simulink model "PE_V2_0"  (R2020b)
settings: Solver=VariableStepAuto  StartTime=0.0  StopTime=10.0  RelTol=1e-3
undefined symbols (not defined in the file): ZERO
libraries: hdlsllib x35, simulink x28, visionhdlutilities x12
(part 3 of 3)

== system PE_V2_0/2DCov PEV1.1/MaxPooling/OutValidGen ==
  ctrl : Inport
  Window_Width : Inport  Port=2
  Feature_Height : Inport  Port=3
  Compare To Constant : simulink/Logic and Bit Operations/Compare To Constant  Commented=on  relop=>  const=0  OutDataTypeStr=boolean
  Constant : Constant  OutDataTypeStr=uint32  SampleTime=-1
  Delay36 : Delay  DelayLength=1
  Logical Operator1 : Logic  Operator=NOT  AllPortsSameDT=off  OutDataTypeStr=boolean
  Logical Operator3 : Logic  Inputs=3  AllPortsSameDT=off  OutDataTypeStr=boolean
  Logical Operator4 : Logic  Operator=NOT  AllPortsSameDT=off  OutDataTypeStr=boolean
  Logical Operator5 : Logic  Operator=OR  AllPortsSameDT=off  OutDataTypeStr=boolean
  Logical Operator6 : Logic  Operator=NOT  Inputs=3  AllPortsSameDT=off  OutDataTypeStr=boolean
  Minus1 : Sum  Inputs=+-
  Minus2 : Sum  Inputs=+-
  NumRow_Counter : hdlsllib/Sources/HDL Counter  CountType=Free running  CountInit=0  CountStep=1  CountMax=2^15  CountFromType=Initial value  CountFrom=0  CountResetPort=on  CountLoadPort=off  CountEnbPort=on  CountDirPort=off  CountDataType=Unsigned  CountWordLen=32  CountFracLen=0  CountSampTime=1
  Pixel Control Bus Selector : BusSelector  OutputSignals=hStart,hEnd,vStart,vEnd,valid
  Relational Operator1 : RelationalOperator  Operator=<  OutDataTypeStr=boolean  RndMeth=Nearest
  Relational Operator2 : RelationalOperator  Operator=<=  OutDataTypeStr=boolean  RndMeth=Nearest
  Row_Counter : hdlsllib/Sources/HDL Counter  CountType=Free running  CountInit=0  CountStep=1  CountMax=2^15  CountFromType=Initial value  CountFrom=0  CountResetPort=on  CountLoadPort=off  CountEnbPort=on  CountDirPort=off  CountDataType=Unsigned  CountWordLen=32  CountFracLen=0  CountSampTime=1
  Terminator1 : Terminator
  Out1 : Outport
  wires:
  NumRow_Counter/1 -> Relational Operator2/2, Compare To Constant/1
  Pixel Control Bus Selector/1 -> NumRow_Counter/2  "<hStart>"
  Minus2/1 -> Relational Operator2/1
  Relational Operator1/1 -> Logical Operator4/1
  Pixel Control Bus Selector/3 -> Logical Operator5/1  "<vStart>"
  Feature_Height/1 -> Minus2/1
  Minus1/1 -> Relational Operator1/2
  Row_Counter/1 -> Relational Operator1/1
  Pixel Control Bus Selector/5 -> Row_Counter/2, Logical Operator1/1, Logical Operator3/2  "<valid>"
  Window_Width/1 -> Minus1/1
  Pixel Control Bus Selector/2 -> Terminator1/1  "<hEnd>"
  Delay36/1 -> Pixel Control Bus Selector/1
  Constant/1 -> Minus1/2, Minus2/2
  Logical Operator6/1 -> Logical Operator3/1
  Logical Operator5/1 -> NumRow_Counter/1
  Pixel Control Bus Selector/4 -> Logical Operator5/2  "<vEnd>"
  Relational Operator2/1 -> Logical Operator6/1
  Logical Operator1/1 -> Row_Counter/1
  Logical Operator4/1 -> Logical Operator3/3
  Logical Operator3/1 -> Out1/1
  ctrl/1 -> Delay36/1

== system PE_V2_0/2DCov PEV1.1/MaxPooling/window Selector ==
  pixel : Inport
  valid : Inport  Port=2
  step : Inport  Port=3
  Add : Sum  Inputs=+-
  Compare To Zero : simulink/Logic and Bit Operations/Compare To Zero  relop===  OutDataTypeStr=boolean
  Constant : Constant  OutDataTypeStr=uint32
  Delay : Delay
  Delay1 : Delay  DelayLength=1
  Delay36 : Delay  DelayLength=1
  Logical Operator : Logic  Operator=NOT  AllPortsSameDT=off  OutDataTypeStr=boolean
  Logical Operator1 : Logic  Operator=OR  AllPortsSameDT=off  OutDataTypeStr=boolean
  Logical Operator2 : Logic  AllPortsSameDT=off  OutDataTypeStr=boolean
  Relational Operator : RelationalOperator  OutDataTypeStr=boolean  RndMeth=Nearest
  Selector1 : Selector  InputPortWidth=2  IndexOptions=Index vector (dialog)  Indices=[1]  OutputSizes=1
  Selector2 : Selector  InputPortWidth=2  IndexOptions=Index vector (dialog)  Indices=[2]  OutputSizes=1
  Selector3 : Selector  InputPortWidth=2  IndexOptions=Index vector (dialog)  Indices=[1]  OutputSizes=1
  Selector4 : Selector  InputPortWidth=2  IndexOptions=Index vector (dialog)  Indices=[2]  OutputSizes=1
  Step Counter : hdlsllib/Sources/HDL Counter  CountType=Free running  CountInit=0  CountStep=1  CountMax=2^15  CountFromType=Initial value  CountFrom=0  CountResetPort=on  CountLoadPort=off  CountEnbPort=on  CountDirPort=off  CountDataType=Unsigned  CountWordLen=32  CountFracLen=0  CountSampTime=1
  Out1 : Outport
  Out2 : Outport  Port=2
  Out3 : Outport  Port=3
  Out4 : Outport  Port=4
  Valid : Outport  Port=5
  wires:
  Selector2/1 -> Out2/1
  Delay/1 -> Selector4/1, Selector3/1
  Selector3/1 -> Out3/1
  Selector1/1 -> Out1/1
  Selector4/1 -> Out4/1
  pixel/1 -> Delay36/1, Delay/1
  Step Counter/1 -> Compare To Zero/1, Relational Operator/1
  Delay1/1 -> Logical Operator2/2, Step Counter/2, Logical Operator/1
  Logical Operator/1 -> Logical Operator1/2
  step/1 -> Add/1
  Constant/1 -> Add/2
  Add/1 -> Relational Operator/2
  Relational Operator/1 -> Logical Operator1/1
  Logical Operator1/1 -> Step Counter/1
  Compare To Zero/1 -> Logical Operator2/1
  Logical Operator2/1 -> Valid/1
  Delay36/1 -> Selector2/1, Selector1/1
  valid/1 -> Delay1/1

== system PE_V2_0/2DConvPE1 V1.5/FUNCTION/Subsystem1/LIne Buffer ==
  Stream_In : Inport
  Stream_Valid : Inport  Port=2
  Weight_Width : Inport  Port=3
  Feature_Area : Inport  Port=4
  Feature_Width : Inport  Port=5
  Feature_Height : Inport  Port=6
  Delay2 : Delay  DelayLength=1
  Line Buffer : Subsystem
  OutValidGen : Subsystem
  Terminator : Terminator
  pixel : Outport
  valid : Outport  Port=2
  wires:
  Feature_Area/1 -> Line Buffer/3(Feature_Area)
  Feature_Height/1 -> OutValidGen/3(Feature_Height)
  Line Buffer/3(shftEnable) -> Terminator/1
  Stream_In/1 -> Line Buffer/1(Stream_In)
  Line Buffer/1(pixel) -> Delay2/1
  Line Buffer/2(ctrl) -> OutValidGen/1(In1)
  Feature_Width/1 -> Line Buffer/4(Feature_Width)
  Stream_Valid/1 -> Line Buffer/2(Stream_Valid)
  Weight_Width/1 -> OutValidGen/2(Weight_Width)
  OutValidGen/1(valid) -> valid/1
  Delay2/1 -> pixel/1

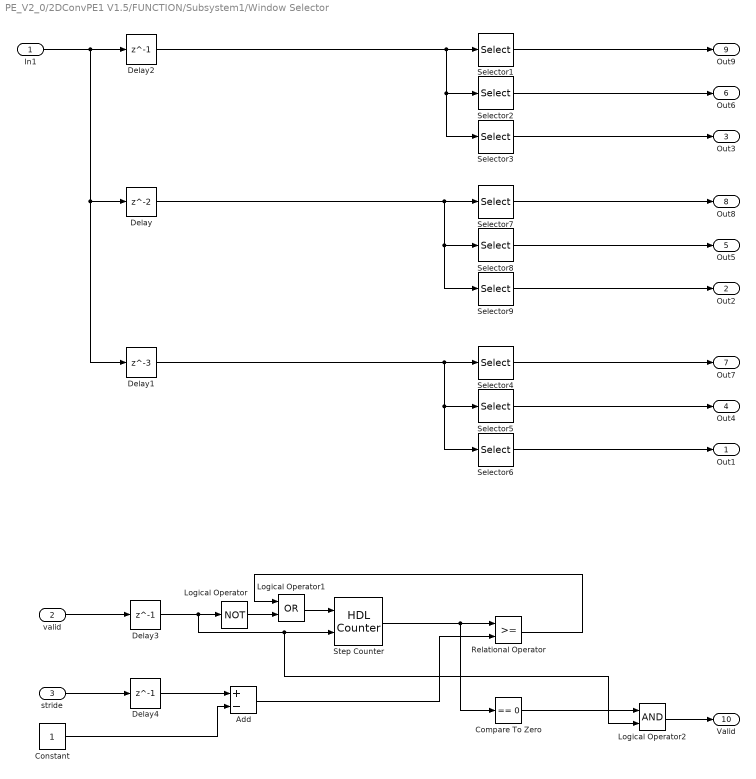
== system PE_V2_0/2DConvPE1 V1.5/FUNCTION/Subsystem1/Window Selector ==
  In1 : Inport
  valid : Inport  Port=2
  stride : Inport  Port=3
  Add : Sum  Inputs=+-
  Compare To Zero : simulink/Logic and Bit Operations/Compare To Zero  relop===  OutDataTypeStr=boolean
  Constant : Constant  OutDataTypeStr=uint32
  Delay : Delay
  Delay1 : Delay  DelayLength=3
  Delay2 : Delay  DelayLength=1
  Delay3 : Delay  DelayLength=1
  Delay4 : Delay  DelayLength=1
  Logical Operator : Logic  Operator=NOT  AllPortsSameDT=off  OutDataTypeStr=boolean
  Logical Operator1 : Logic  Operator=OR  AllPortsSameDT=off  OutDataTypeStr=boolean
  Logical Operator2 : Logic  AllPortsSameDT=off  OutDataTypeStr=boolean
  Relational Operator : RelationalOperator  OutDataTypeStr=boolean  RndMeth=Nearest
  Selector1 : Selector  InputPortWidth=3  IndexOptions=Index vector (dialog)  Indices=[1]  OutputSizes=1
  Selector2 : Selector  InputPortWidth=3  IndexOptions=Index vector (dialog)  Indices=[2]  OutputSizes=1
  Selector3 : Selector  InputPortWidth=3  IndexOptions=Index vector (dialog)  Indices=[3]  OutputSizes=1
  Selector4 : Selector  InputPortWidth=3  IndexOptions=Index vector (dialog)  Indices=[1]  OutputSizes=1
  Selector5 : Selector  InputPortWidth=3  IndexOptions=Index vector (dialog)  Indices=[2]  OutputSizes=1
  Selector6 : Selector  InputPortWidth=3  IndexOptions=Index vector (dialog)  Indices=[3]  OutputSizes=1
  Selector7 : Selector  InputPortWidth=3  IndexOptions=Index vector (dialog)  Indices=[1]  OutputSizes=1
  Selector8 : Selector  InputPortWidth=3  IndexOptions=Index vector (dialog)  Indices=[2]  OutputSizes=1
  Selector9 : Selector  InputPortWidth=3  IndexOptions=Index vector (dialog)  Indices=[3]  OutputSizes=1
  Step Counter : hdlsllib/Sources/HDL Counter  CountType=Free running  CountInit=0  CountStep=1  CountMax=2^15  CountFromType=Initial value  CountFrom=0  CountResetPort=on  CountLoadPort=off  CountEnbPort=on  CountDirPort=off  CountDataType=Unsigned  CountWordLen=32  CountFracLen=0  CountSampTime=1
  Out1 : Outport
  Out2 : Outport  Port=2
  Out3 : Outport  Port=3
  Out4 : Outport  Port=4
  Out5 : Outport  Port=5
  Out6 : Outport  Port=6
  Out7 : Outport  Port=7
  Out8 : Outport  Port=8
  Out9 : Outport  Port=9
  Valid : Outport  Port=10
  wires:
  In1/1 -> Delay2/1, Delay1/1, Delay/1
  Selector9/1 -> Out2/1
  Delay/1 -> Selector9/1, Selector8/1, Selector7/1
  Selector5/1 -> Out4/1
  Selector6/1 -> Out1/1
  Selector4/1 -> Out7/1
  Delay1/1 -> Selector6/1, Selector5/1, Selector4/1
  Relational Operator/1 -> Logical Operator1/1
  Constant/1 -> Add/2
  Logical Operator2/1 -> Valid/1
  Compare To Zero/1 -> Logical Operator2/1
  Logical Operator1/1 -> Step Counter/1
  Logical Operator/1 -> Logical Operator1/2
  Delay4/1 -> Add/1
  Step Counter/1 -> Compare To Zero/1, Relational Operator/1
  Delay3/1 -> Logical Operator2/2, Step Counter/2, Logical Operator/1
  Add/1 -> Relational Operator/2
  Delay2/1 -> Selector3/1, Selector2/1, Selector1/1
  valid/1 -> Delay3/1
  stride/1 -> Delay4/1
  Selector8/1 -> Out5/1
  Selector7/1 -> Out8/1
  Selector3/1 -> Out3/1
  Selector2/1 -> Out6/1
  Selector1/1 -> Out9/1

== system PE_V2_0/2DConvPE1 V1.5/FUNCTION/Subsystem1/weight_register ==
  In1 : Inport
  Enable : EnablePort
  Delay{1,3..8,40} (8 alike) : Delay  DelayLength=1
  Out2 : Outport
  Out3 : Outport  Port=2
  Out4 : Outport  Port=3
  Out5 : Outport  Port=4
  Out6 : Outport  Port=5
  Out7 : Outport  Port=6
  Out8 : Outport  Port=7
  Out9 : Outport  Port=8
  Out1 : Outport  Port=9
  wires:
  Delay40/1 -> Delay7/1, Out9/1
  In1/1 -> Out1/1, Delay40/1
  Delay7/1 -> Out8/1, Delay1/1
  Delay1/1 -> Out7/1, Delay5/1
  Delay5/1 -> Out6/1, Delay8/1
  Delay8/1 -> Out5/1, Delay6/1
  Delay6/1 -> Out4/1, Delay4/1
  Delay4/1 -> Out3/1, Delay3/1
  Delay3/1 -> Out2/1

== system PE_V2_0/2DConvPE1 V1.5/MaxPooling/Line Buffer1/CtrlGen ==
  note: valid
  note: vEnd
  note: vStart
  note: hEnd
  note: hstart
  Stream_In : Inport
  Stream_Valid : Inport  Port=2
  Feature_Area : Inport  Port=3
  Feature_Width : Inport  Port=4
  Compare To Zero : simulink/Logic and Bit Operations/Compare To Zero  relop===  OutDataTypeStr=boolean
  Compare To Zero1 : simulink/Logic and Bit Operations/Compare To Zero  relop===  OutDataTypeStr=boolean
  Constant : Constant  OutDataTypeStr=uint32  SampleTime=-1
  Constant1 : Constant  OutDataTypeStr=uint32  SampleTime=-1
  Delay1 : Delay  DelayLength=1
  Delay36 : Delay  DelayLength=1
  Feature Area Counter : hdlsllib/Sources/HDL Counter  CountType=Free running  CountInit=0  CountStep=1  CountMax=2^15  CountFromType=Initial value  CountFrom=0  CountResetPort=on  CountLoadPort=off  CountEnbPort=on  CountDirPort=off  CountDataType=Unsigned  CountWordLen=32  CountFracLen=0  CountSampTime=1
  Feature Row Counter : hdlsllib/Sources/HDL Counter  CountType=Free running  CountInit=0  CountStep=1  CountMax=2^15  CountFromType=Initial value  CountFrom=0  CountResetPort=on  CountLoadPort=off  CountEnbPort=on  CountDirPort=off  CountDataType=Unsigned  CountWordLen=32  CountFracLen=0  CountSampTime=1
  Logical Operator : Logic  Operator=OR  AllPortsSameDT=off  OutDataTypeStr=boolean
  Logical Operator{1..3,5} (4 alike) : Logic  AllPortsSameDT=off  OutDataTypeStr=boolean
  Minus1 : Sum  Inputs=+-
  Minus2 : Sum  Inputs=+-
  Pixel Control Bus Creator : visionhdlutilities/Pixel Control Bus Creator
      settings: SourceProductBaseCode=VT
  Relational Operator1 : RelationalOperator  Operator===  OutDataTypeStr=boolean  RndMeth=Nearest
  Relational Operator2 : RelationalOperator  Operator===  OutDataTypeStr=boolean  RndMeth=Nearest
  Relational Operator3 : RelationalOperator  Operator===  OutDataTypeStr=boolean  RndMeth=Nearest
  StreamOut : Outport
  Ctrl : Outport  Port=2
  wires:
  Minus2/1 -> Relational Operator3/2, Relational Operator2/2
  Feature Row Counter/1 -> Relational Operator2/1, Relational Operator3/1, Compare To Zero/1
  Relational Operator2/1 -> Feature Row Counter/1
  Compare To Zero/1 -> Logical Operator/2
  Relational Operator3/1 -> Logical Operator2/1
  Feature_Area/1 -> Minus1/1
  Constant/1 -> Minus1/2
  Logical Operator/1 -> Logical Operator1/1
  Constant1/1 -> Minus2/2
  Feature_Width/1 -> Minus2/1
  Pixel Control Bus Creator/1 -> Ctrl/1
  Delay1/1 -> Feature Area Counter/2, Feature Row Counter/2, Logical Operator5/2, Logical Operator2/2, Logical Operator1/2, Logical Operator3/2, Pixel Control Bus Creator/5
  Delay36/1 -> StreamOut/1
  Logical Operator1/1 -> Pixel Control Bus Creator/1
  Logical Operator2/1 -> Pixel Control Bus Creator/2
  Logical Operator3/1 -> Pixel Control Bus Creator/4
  Logical Operator5/1 -> Pixel Control Bus Creator/3
  Feature Area Counter/1 -> Compare To Zero1/1, Relational Operator1/1
  Minus1/1 -> Relational Operator1/2
  Relational Operator1/1 -> Feature Area Counter/1, Logical Operator3/1
  Compare To Zero1/1 -> Logical Operator/1, Logical Operator5/1
  Stream_In/1 -> Delay36/1
  Stream_Valid/1 -> Delay1/1

== system PE_V2_0/2DConvPE1 V2.0/Line Buffer/LIne Buffer/Line Buffer ==
  Stream_In : Inport
  Stream_Valid : Inport  Port=2
  Feature_Area : Inport  Port=3
  Feature_Width : Inport  Port=4
  CtrlGen : Subsystem
  Line Buffer : visionhdlutilities/Line Buffer  NeighborhoodSize=[3 1]  PaddingMethod=Constant  PaddingValue=0  LineBufferSize=128  SimulateUsing=Code generation
      settings: SourceProductBaseCode=VT
  pixel : Outport
  ctrl : Outport  Port=2
  shftEnable : Outport  Port=3
  wires:
  Feature_Area/1 -> CtrlGen/3(Feature_Area)
  Line Buffer/2 -> ctrl/1
  CtrlGen/1(StreamOut) -> Line Buffer/1
  Feature_Width/1 -> CtrlGen/4(Feature_Width)
  Stream_In/1 -> CtrlGen/1(Stream_In)
  CtrlGen/2(Ctrl) -> Line Buffer/2
  Stream_Valid/1 -> CtrlGen/2(Stream_Valid)
  Line Buffer/3 -> shftEnable/1
  Line Buffer/1 -> pixel/1

== system PE_V2_0/2DConvPE1 V2.0/Line Buffer/LIne Buffer/OutValidGen ==
  In1 : Inport
  Weight_Width : Inport  Port=2
  Feature_Height : Inport  Port=3
  Compare To Constant : simulink/Logic and Bit Operations/Compare To Constant  relop=>  const=0  OutDataTypeStr=boolean
  Constant : Constant  OutDataTypeStr=uint32  SampleTime=-1
  Delay2 : Delay  DelayLength=1
  Logical Operator1 : Logic  Operator=NOT  AllPortsSameDT=off  OutDataTypeStr=boolean
  Logical Operator2 : Logic  Operator=OR  AllPortsSameDT=off  OutDataTypeStr=boolean
  Logical Operator3 : Logic  Inputs=4  AllPortsSameDT=off  OutDataTypeStr=boolean
  Logical Operator4 : Logic  Operator=NOT  AllPortsSameDT=off  OutDataTypeStr=boolean
  Logical Operator5 : Logic  Operator=OR  AllPortsSameDT=off  OutDataTypeStr=boolean
  Logical Operator6 : Logic  Operator=NOT  Inputs=3  AllPortsSameDT=off  OutDataTypeStr=boolean
  Minus1 : Sum  Inputs=+--
  Minus2 : Sum  Inputs=+-
  NumRow_Counter : hdlsllib/Sources/HDL Counter  CountType=Free running  CountInit=0  CountStep=1  CountMax=2^15  CountFromType=Initial value  CountFrom=0  CountResetPort=on  CountLoadPort=off  CountEnbPort=on  CountDirPort=off  CountDataType=Unsigned  CountWordLen=32  CountFracLen=0  CountSampTime=1
  Pixel Control Bus Selector : BusSelector  OutputSignals=hStart,hEnd,vStart,vEnd,valid
  Relational Operator1 : RelationalOperator  Operator=<  OutDataTypeStr=boolean  RndMeth=Nearest
  Relational Operator2 : RelationalOperator  Operator=<=  OutDataTypeStr=boolean  RndMeth=Nearest
  Row_Counter : hdlsllib/Sources/HDL Counter  CountType=Free running  CountInit=0  CountStep=1  CountMax=2^15  CountFromType=Initial value  CountFrom=0  CountResetPort=on  CountLoadPort=off  CountEnbPort=on  CountDirPort=off  CountDataType=Unsigned  CountWordLen=32  CountFracLen=0  CountSampTime=1
  Terminator1 : Terminator
  valid : Outport
  wires:
  Compare To Constant/1 -> Logical Operator3/2
  NumRow_Counter/1 -> Relational Operator2/2, Compare To Constant/1
  Pixel Control Bus Selector/1 -> NumRow_Counter/2, Logical Operator2/1  "<hStart>"
  Minus2/1 -> Relational Operator2/1
  Relational Operator1/1 -> Logical Operator4/1
  Logical Operator1/1 -> Logical Operator2/2
  Pixel Control Bus Selector/3 -> Logical Operator5/1  "<vStart>"
  Feature_Height/1 -> Minus2/1
  Minus1/1 -> Relational Operator1/2
  Row_Counter/1 -> Relational Operator1/1
  Pixel Control Bus Selector/5 -> Logical Operator1/1, Row_Counter/2, Logical Operator3/3  "<valid>"
  Weight_Width/1 -> Minus1/1
  Pixel Control Bus Selector/2 -> Terminator1/1  "<hEnd>"
  Delay2/1 -> Pixel Control Bus Selector/1
  Constant/1 -> Minus1/3, Minus1/2, Minus2/2
  Logical Operator6/1 -> Logical Operator3/1
  Logical Operator5/1 -> NumRow_Counter/1
  Pixel Control Bus Selector/4 -> Logical Operator5/2  "<vEnd>"
  Relational Operator2/1 -> Logical Operator6/1
  Logical Operator2/1 -> Row_Counter/1
  Logical Operator4/1 -> Logical Operator3/4
  Logical Operator3/1 -> valid/1
  In1/1 -> Delay2/1

== system PE_V2_0/2DConvPE1 V2.0/MaxPooling/Line Buffer1/CtrlGen ==
  note: valid
  note: vEnd
  note: vStart
  note: hEnd
  note: hstart
  Stream_In : Inport
  Stream_Valid : Inport  Port=2
  Feature_Area : Inport  Port=3
  Feature_Width : Inport  Port=4
  Compare To Zero : simulink/Logic and Bit Operations/Compare To Zero  relop===  OutDataTypeStr=boolean
  Compare To Zero1 : simulink/Logic and Bit Operations/Compare To Zero  relop===  OutDataTypeStr=boolean
  Constant : Constant  OutDataTypeStr=uint32  SampleTime=-1
  Constant1 : Constant  OutDataTypeStr=uint32  SampleTime=-1
  Delay1 : Delay  DelayLength=1
  Delay36 : Delay  DelayLength=1
  Feature Area Counter : hdlsllib/Sources/HDL Counter  CountType=Free running  CountInit=0  CountStep=1  CountMax=2^15  CountFromType=Initial value  CountFrom=0  CountResetPort=on  CountLoadPort=off  CountEnbPort=on  CountDirPort=off  CountDataType=Unsigned  CountWordLen=32  CountFracLen=0  CountSampTime=1
  Feature Row Counter : hdlsllib/Sources/HDL Counter  CountType=Free running  CountInit=0  CountStep=1  CountMax=2^15  CountFromType=Initial value  CountFrom=0  CountResetPort=on  CountLoadPort=off  CountEnbPort=on  CountDirPort=off  CountDataType=Unsigned  CountWordLen=32  CountFracLen=0  CountSampTime=1
  Logical Operator : Logic  Operator=OR  AllPortsSameDT=off  OutDataTypeStr=boolean
  Logical Operator{1..3,5} (4 alike) : Logic  AllPortsSameDT=off  OutDataTypeStr=boolean
  Minus1 : Sum  Inputs=+-
  Minus2 : Sum  Inputs=+-
  Pixel Control Bus Creator : visionhdlutilities/Pixel Control Bus Creator
      settings: SourceProductBaseCode=VT
  Relational Operator1 : RelationalOperator  Operator===  OutDataTypeStr=boolean  RndMeth=Nearest
  Relational Operator2 : RelationalOperator  Operator===  OutDataTypeStr=boolean  RndMeth=Nearest
  Relational Operator3 : RelationalOperator  Operator===  OutDataTypeStr=boolean  RndMeth=Nearest
  StreamOut : Outport
  Ctrl : Outport  Port=2
  wires:
  Minus2/1 -> Relational Operator3/2, Relational Operator2/2
  Feature Row Counter/1 -> Relational Operator2/1, Relational Operator3/1, Compare To Zero/1
  Relational Operator2/1 -> Feature Row Counter/1
  Compare To Zero/1 -> Logical Operator/2
  Relational Operator3/1 -> Logical Operator2/1
  Feature_Area/1 -> Minus1/1
  Constant/1 -> Minus1/2
  Logical Operator/1 -> Logical Operator1/1
  Constant1/1 -> Minus2/2
  Feature_Width/1 -> Minus2/1
  Pixel Control Bus Creator/1 -> Ctrl/1
  Delay1/1 -> Feature Area Counter/2, Feature Row Counter/2, Logical Operator5/2, Logical Operator2/2, Logical Operator1/2, Logical Operator3/2, Pixel Control Bus Creator/5
  Delay36/1 -> StreamOut/1
  Logical Operator1/1 -> Pixel Control Bus Creator/1
  Logical Operator2/1 -> Pixel Control Bus Creator/2
  Logical Operator3/1 -> Pixel Control Bus Creator/4
  Logical Operator5/1 -> Pixel Control Bus Creator/3
  Feature Area Counter/1 -> Compare To Zero1/1, Relational Operator1/1
  Minus1/1 -> Relational Operator1/2
  Relational Operator1/1 -> Feature Area Counter/1, Logical Operator3/1
  Compare To Zero1/1 -> Logical Operator/1, Logical Operator5/1
  Stream_In/1 -> Delay36/1
  Stream_Valid/1 -> Delay1/1

== system PE_V2_0/2DCov PEV1.1/LIne Buffer/Line Buffer/CtrlGen ==
  note: valid
  note: vEnd
  note: vStart
  note: hEnd
  note: hstart
  Stream_In : Inport
  Stream_Valid : Inport  Port=2
  Feature_Area : Inport  Port=3
  Feature_Width : Inport  Port=4
  Compare To Zero : simulink/Logic and Bit Operations/Compare To Zero  relop===  OutDataTypeStr=boolean
  Compare To Zero1 : simulink/Logic and Bit Operations/Compare To Zero  relop===  OutDataTypeStr=boolean
  Constant : Constant  OutDataTypeStr=uint32  SampleTime=-1
  Constant1 : Constant  OutDataTypeStr=uint32  SampleTime=-1
  Delay3 : Delay  DelayLength=1
  Delay35 : Delay  DelayLength=1
  Feature Area Counter : hdlsllib/Sources/HDL Counter  CountType=Free running  CountInit=0  CountStep=1  CountMax=2^15  CountFromType=Initial value  CountFrom=0  CountResetPort=on  CountLoadPort=off  CountEnbPort=on  CountDirPort=off  CountDataType=Unsigned  CountWordLen=32  CountFracLen=0  CountSampTime=1
  Feature Row Counter : hdlsllib/Sources/HDL Counter  CountType=Free running  CountInit=0  CountStep=1  CountMax=2^15  CountFromType=Initial value  CountFrom=0  CountResetPort=on  CountLoadPort=off  CountEnbPort=on  CountDirPort=off  CountDataType=Unsigned  CountWordLen=32  CountFracLen=0  CountSampTime=1
  Logical Operator : Logic  Operator=OR  AllPortsSameDT=off  OutDataTypeStr=boolean
  Logical Operator{1..3,5} (4 alike) : Logic  AllPortsSameDT=off  OutDataTypeStr=boolean
  Minus1 : Sum  Inputs=+-
  Minus2 : Sum  Inputs=+-
  Pixel Control Bus Creator : visionhdlutilities/Pixel Control Bus Creator
      settings: SourceProductBaseCode=VT
  Relational Operator1 : RelationalOperator  Operator===  OutDataTypeStr=boolean  RndMeth=Nearest
  Relational Operator2 : RelationalOperator  Operator===  OutDataTypeStr=boolean  RndMeth=Nearest
  Relational Operator3 : RelationalOperator  Operator===  OutDataTypeStr=boolean  RndMeth=Nearest
  StreamOut : Outport
  Ctrl : Outport  Port=2
  wires:
  Minus2/1 -> Relational Operator3/2, Relational Operator2/2
  Feature Row Counter/1 -> Relational Operator2/1, Relational Operator3/1, Compare To Zero/1
  Relational Operator2/1 -> Feature Row Counter/1
  Compare To Zero/1 -> Logical Operator/2
  Relational Operator3/1 -> Logical Operator2/1
  Feature_Area/1 -> Minus1/1
  Constant/1 -> Minus1/2
  Logical Operator/1 -> Logical Operator1/1
  Constant1/1 -> Minus2/2
  Feature_Width/1 -> Minus2/1
  Pixel Control Bus Creator/1 -> Ctrl/1
  Delay3/1 -> Feature Area Counter/2, Feature Row Counter/2, Logical Operator5/2, Logical Operator2/2, Logical Operator1/2, Logical Operator3/2, Pixel Control Bus Creator/5
  Stream_In/1 -> Delay35/1
  Logical Operator1/1 -> Pixel Control Bus Creator/1
  Logical Operator2/1 -> Pixel Control Bus Creator/2
  Logical Operator3/1 -> Pixel Control Bus Creator/4
  Logical Operator5/1 -> Pixel Control Bus Creator/3
  Feature Area Counter/1 -> Compare To Zero1/1, Relational Operator1/1
  Minus1/1 -> Relational Operator1/2
  Relational Operator1/1 -> Feature Area Counter/1, Logical Operator3/1
  Compare To Zero1/1 -> Logical Operator/1, Logical Operator5/1
  Delay35/1 -> StreamOut/1
  Stream_Valid/1 -> Delay3/1

== system PE_V2_0/2DCov PEV1.1/MaxPooling/Line Buffer1/CtrlGen ==
  note: valid
  note: vEnd
  note: vStart
  note: hEnd
  note: hstart
  Stream_In : Inport
  Stream_Valid : Inport  Port=2
  Feature_Area : Inport  Port=3
  Feature_Width : Inport  Port=4
  Compare To Zero : simulink/Logic and Bit Operations/Compare To Zero  relop===  OutDataTypeStr=boolean
  Compare To Zero1 : simulink/Logic and Bit Operations/Compare To Zero  relop===  OutDataTypeStr=boolean
  Constant : Constant  OutDataTypeStr=uint32  SampleTime=-1
  Constant1 : Constant  OutDataTypeStr=uint32  SampleTime=-1
  Delay1 : Delay  DelayLength=1
  Delay36 : Delay  DelayLength=1
  Feature Area Counter : hdlsllib/Sources/HDL Counter  CountType=Free running  CountInit=0  CountStep=1  CountMax=2^15  CountFromType=Initial value  CountFrom=0  CountResetPort=on  CountLoadPort=off  CountEnbPort=on  CountDirPort=off  CountDataType=Unsigned  CountWordLen=32  CountFracLen=0  CountSampTime=1
  Feature Row Counter : hdlsllib/Sources/HDL Counter  CountType=Free running  CountInit=0  CountStep=1  CountMax=2^15  CountFromType=Initial value  CountFrom=0  CountResetPort=on  CountLoadPort=off  CountEnbPort=on  CountDirPort=off  CountDataType=Unsigned  CountWordLen=32  CountFracLen=0  CountSampTime=1
  Logical Operator : Logic  Operator=OR  AllPortsSameDT=off  OutDataTypeStr=boolean
  Logical Operator{1..3,5} (4 alike) : Logic  AllPortsSameDT=off  OutDataTypeStr=boolean
  Minus1 : Sum  Inputs=+-
  Minus2 : Sum  Inputs=+-
  Pixel Control Bus Creator : visionhdlutilities/Pixel Control Bus Creator
      settings: SourceProductBaseCode=VT
  Relational Operator1 : RelationalOperator  Operator===  OutDataTypeStr=boolean  RndMeth=Nearest
  Relational Operator2 : RelationalOperator  Operator===  OutDataTypeStr=boolean  RndMeth=Nearest
  Relational Operator3 : RelationalOperator  Operator===  OutDataTypeStr=boolean  RndMeth=Nearest
  StreamOut : Outport
  Ctrl : Outport  Port=2
  wires:
  Minus2/1 -> Relational Operator3/2, Relational Operator2/2
  Feature Row Counter/1 -> Relational Operator2/1, Relational Operator3/1, Compare To Zero/1
  Relational Operator2/1 -> Feature Row Counter/1
  Compare To Zero/1 -> Logical Operator/2
  Relational Operator3/1 -> Logical Operator2/1
  Feature_Area/1 -> Minus1/1
  Constant/1 -> Minus1/2
  Logical Operator/1 -> Logical Operator1/1
  Constant1/1 -> Minus2/2
  Feature_Width/1 -> Minus2/1
  Pixel Control Bus Creator/1 -> Ctrl/1
  Delay1/1 -> Feature Area Counter/2, Feature Row Counter/2, Logical Operator5/2, Logical Operator2/2, Logical Operator1/2, Logical Operator3/2, Pixel Control Bus Creator/5
  Delay36/1 -> StreamOut/1
  Logical Operator1/1 -> Pixel Control Bus Creator/1
  Logical Operator2/1 -> Pixel Control Bus Creator/2
  Logical Operator3/1 -> Pixel Control Bus Creator/4
  Logical Operator5/1 -> Pixel Control Bus Creator/3
  Feature Area Counter/1 -> Compare To Zero1/1, Relational Operator1/1
  Minus1/1 -> Relational Operator1/2
  Relational Operator1/1 -> Feature Area Counter/1, Logical Operator3/1
  Compare To Zero1/1 -> Logical Operator/1, Logical Operator5/1
  Stream_In/1 -> Delay36/1
  Stream_Valid/1 -> Delay1/1

== system PE_V2_0/2DConvPE1 V1.5/FUNCTION/Subsystem1/LIne Buffer/Line Buffer ==
  Stream_In : Inport
  Stream_Valid : Inport  Port=2
  Feature_Area : Inport  Port=3
  Feature_Width : Inport  Port=4
  CtrlGen : Subsystem
  Line Buffer : visionhdlutilities/Line Buffer  NeighborhoodSize=[3 1]  PaddingMethod=Constant  PaddingValue=0  LineBufferSize=128  SimulateUsing=Code generation
      settings: SourceProductBaseCode=VT
  pixel : Outport
  ctrl : Outport  Port=2
  shftEnable : Outport  Port=3
  wires:
  Feature_Area/1 -> CtrlGen/3(Feature_Area)
  Line Buffer/2 -> ctrl/1
  CtrlGen/1(StreamOut) -> Line Buffer/1
  Feature_Width/1 -> CtrlGen/4(Feature_Width)
  Stream_In/1 -> CtrlGen/1(Stream_In)
  CtrlGen/2(Ctrl) -> Line Buffer/2
  Stream_Valid/1 -> CtrlGen/2(Stream_Valid)
  Line Buffer/3 -> shftEnable/1
  Line Buffer/1 -> pixel/1

== system PE_V2_0/2DConvPE1 V1.5/FUNCTION/Subsystem1/LIne Buffer/OutValidGen ==
  In1 : Inport
  Weight_Width : Inport  Port=2
  Feature_Height : Inport  Port=3
  Compare To Constant : simulink/Logic and Bit Operations/Compare To Constant  relop=>  const=0  OutDataTypeStr=boolean
  Constant : Constant  OutDataTypeStr=uint32  SampleTime=-1
  Delay2 : Delay  DelayLength=1
  Logical Operator1 : Logic  Operator=NOT  AllPortsSameDT=off  OutDataTypeStr=boolean
  Logical Operator2 : Logic  Operator=OR  AllPortsSameDT=off  OutDataTypeStr=boolean
  Logical Operator3 : Logic  Inputs=4  AllPortsSameDT=off  OutDataTypeStr=boolean
  Logical Operator4 : Logic  Operator=NOT  AllPortsSameDT=off  OutDataTypeStr=boolean
  Logical Operator5 : Logic  Operator=OR  AllPortsSameDT=off  OutDataTypeStr=boolean
  Logical Operator6 : Logic  Operator=NOT  Inputs=3  AllPortsSameDT=off  OutDataTypeStr=boolean
  Minus1 : Sum  Inputs=+--
  Minus2 : Sum  Inputs=+-
  NumRow_Counter : hdlsllib/Sources/HDL Counter  CountType=Free running  CountInit=0  CountStep=1  CountMax=2^15  CountFromType=Initial value  CountFrom=0  CountResetPort=on  CountLoadPort=off  CountEnbPort=on  CountDirPort=off  CountDataType=Unsigned  CountWordLen=32  CountFracLen=0  CountSampTime=1
  Pixel Control Bus Selector : BusSelector  OutputSignals=hStart,hEnd,vStart,vEnd,valid
  Relational Operator1 : RelationalOperator  Operator=<  OutDataTypeStr=boolean  RndMeth=Nearest
  Relational Operator2 : RelationalOperator  Operator=<=  OutDataTypeStr=boolean  RndMeth=Nearest
  Row_Counter : hdlsllib/Sources/HDL Counter  CountType=Free running  CountInit=0  CountStep=1  CountMax=2^15  CountFromType=Initial value  CountFrom=0  CountResetPort=on  CountLoadPort=off  CountEnbPort=on  CountDirPort=off  CountDataType=Unsigned  CountWordLen=32  CountFracLen=0  CountSampTime=1
  Terminator1 : Terminator
  valid : Outport
  wires:
  Compare To Constant/1 -> Logical Operator3/2
  NumRow_Counter/1 -> Relational Operator2/2, Compare To Constant/1
  Pixel Control Bus Selector/1 -> NumRow_Counter/2, Logical Operator2/1  "<hStart>"
  Minus2/1 -> Relational Operator2/1
  Relational Operator1/1 -> Logical Operator4/1
  Logical Operator1/1 -> Logical Operator2/2
  Pixel Control Bus Selector/3 -> Logical Operator5/1  "<vStart>"
  Feature_Height/1 -> Minus2/1
  Minus1/1 -> Relational Operator1/2
  Row_Counter/1 -> Relational Operator1/1
  Pixel Control Bus Selector/5 -> Logical Operator1/1, Row_Counter/2, Logical Operator3/3  "<valid>"
  Weight_Width/1 -> Minus1/1
  Pixel Control Bus Selector/2 -> Terminator1/1  "<hEnd>"
  Delay2/1 -> Pixel Control Bus Selector/1
  Constant/1 -> Minus1/3, Minus1/2, Minus2/2
  Logical Operator6/1 -> Logical Operator3/1
  Logical Operator5/1 -> NumRow_Counter/1
  Pixel Control Bus Selector/4 -> Logical Operator5/2  "<vEnd>"
  Relational Operator2/1 -> Logical Operator6/1
  Logical Operator2/1 -> Row_Counter/1
  Logical Operator4/1 -> Logical Operator3/4
  Logical Operator3/1 -> valid/1
  In1/1 -> Delay2/1

== system PE_V2_0/2DConvPE1 V2.0/Line Buffer/LIne Buffer/Line Buffer/CtrlGen ==
  note: valid
  note: vEnd
  note: vStart
  note: hEnd
  note: hstart
  Stream_In : Inport
  Stream_Valid : Inport  Port=2
  Feature_Area : Inport  Port=3
  Feature_Width : Inport  Port=4
  Compare To Zero : simulink/Logic and Bit Operations/Compare To Zero  relop===  OutDataTypeStr=boolean
  Compare To Zero1 : simulink/Logic and Bit Operations/Compare To Zero  relop===  OutDataTypeStr=boolean
  Constant : Constant  OutDataTypeStr=uint32  SampleTime=-1
  Constant1 : Constant  OutDataTypeStr=uint32  SampleTime=-1
  Delay3 : Delay  DelayLength=1
  Delay35 : Delay  DelayLength=1
  Feature Area Counter : hdlsllib/Sources/HDL Counter  CountType=Free running  CountInit=0  CountStep=1  CountMax=2^15  CountFromType=Initial value  CountFrom=0  CountResetPort=on  CountLoadPort=off  CountEnbPort=on  CountDirPort=off  CountDataType=Unsigned  CountWordLen=32  CountFracLen=0  CountSampTime=1
  Feature Row Counter : hdlsllib/Sources/HDL Counter  CountType=Free running  CountInit=0  CountStep=1  CountMax=2^15  CountFromType=Initial value  CountFrom=0  CountResetPort=on  CountLoadPort=off  CountEnbPort=on  CountDirPort=off  CountDataType=Unsigned  CountWordLen=32  CountFracLen=0  CountSampTime=1
  Logical Operator : Logic  Operator=OR  AllPortsSameDT=off  OutDataTypeStr=boolean
  Logical Operator{1..3,5} (4 alike) : Logic  AllPortsSameDT=off  OutDataTypeStr=boolean
  Minus1 : Sum  Inputs=+-
  Minus2 : Sum  Inputs=+-
  Pixel Control Bus Creator : visionhdlutilities/Pixel Control Bus Creator
      settings: SourceProductBaseCode=VT
  Relational Operator1 : RelationalOperator  Operator===  OutDataTypeStr=boolean  RndMeth=Nearest
  Relational Operator2 : RelationalOperator  Operator===  OutDataTypeStr=boolean  RndMeth=Nearest
  Relational Operator3 : RelationalOperator  Operator===  OutDataTypeStr=boolean  RndMeth=Nearest
  StreamOut : Outport
  Ctrl : Outport  Port=2
  wires:
  Minus2/1 -> Relational Operator3/2, Relational Operator2/2
  Feature Row Counter/1 -> Relational Operator2/1, Relational Operator3/1, Compare To Zero/1
  Relational Operator2/1 -> Feature Row Counter/1
  Compare To Zero/1 -> Logical Operator/2
  Relational Operator3/1 -> Logical Operator2/1
  Feature_Area/1 -> Minus1/1
  Constant/1 -> Minus1/2
  Logical Operator/1 -> Logical Operator1/1
  Constant1/1 -> Minus2/2
  Feature_Width/1 -> Minus2/1
  Pixel Control Bus Creator/1 -> Ctrl/1
  Delay3/1 -> Feature Area Counter/2, Feature Row Counter/2, Logical Operator5/2, Logical Operator2/2, Logical Operator1/2, Logical Operator3/2, Pixel Control Bus Creator/5
  Stream_In/1 -> Delay35/1
  Logical Operator1/1 -> Pixel Control Bus Creator/1
  Logical Operator2/1 -> Pixel Control Bus Creator/2
  Logical Operator3/1 -> Pixel Control Bus Creator/4
  Logical Operator5/1 -> Pixel Control Bus Creator/3
  Feature Area Counter/1 -> Compare To Zero1/1, Relational Operator1/1
  Minus1/1 -> Relational Operator1/2
  Relational Operator1/1 -> Feature Area Counter/1, Logical Operator3/1
  Compare To Zero1/1 -> Logical Operator/1, Logical Operator5/1
  Delay35/1 -> StreamOut/1
  Stream_Valid/1 -> Delay3/1

== system PE_V2_0/2DConvPE1 V1.5/FUNCTION/Subsystem1/LIne Buffer/Line Buffer/CtrlGen ==
  note: valid
  note: vEnd
  note: vStart
  note: hEnd
  note: hstart
  Stream_In : Inport
  Stream_Valid : Inport  Port=2
  Feature_Area : Inport  Port=3
  Feature_Width : Inport  Port=4
  Compare To Zero : simulink/Logic and Bit Operations/Compare To Zero  relop===  OutDataTypeStr=boolean
  Compare To Zero1 : simulink/Logic and Bit Operations/Compare To Zero  relop===  OutDataTypeStr=boolean
  Constant : Constant  OutDataTypeStr=uint32  SampleTime=-1
  Constant1 : Constant  OutDataTypeStr=uint32  SampleTime=-1
  Delay3 : Delay  DelayLength=1
  Delay35 : Delay  DelayLength=1
  Feature Area Counter : hdlsllib/Sources/HDL Counter  CountType=Free running  CountInit=0  CountStep=1  CountMax=2^15  CountFromType=Initial value  CountFrom=0  CountResetPort=on  CountLoadPort=off  CountEnbPort=on  CountDirPort=off  CountDataType=Unsigned  CountWordLen=32  CountFracLen=0  CountSampTime=1
  Feature Row Counter : hdlsllib/Sources/HDL Counter  CountType=Free running  CountInit=0  CountStep=1  CountMax=2^15  CountFromType=Initial value  CountFrom=0  CountResetPort=on  CountLoadPort=off  CountEnbPort=on  CountDirPort=off  CountDataType=Unsigned  CountWordLen=32  CountFracLen=0  CountSampTime=1
  Logical Operator : Logic  Operator=OR  AllPortsSameDT=off  OutDataTypeStr=boolean
  Logical Operator{1..3,5} (4 alike) : Logic  AllPortsSameDT=off  OutDataTypeStr=boolean
  Minus1 : Sum  Inputs=+-
  Minus2 : Sum  Inputs=+-
  Pixel Control Bus Creator : visionhdlutilities/Pixel Control Bus Creator
      settings: SourceProductBaseCode=VT
  Relational Operator1 : RelationalOperator  Operator===  OutDataTypeStr=boolean  RndMeth=Nearest
  Relational Operator2 : RelationalOperator  Operator===  OutDataTypeStr=boolean  RndMeth=Nearest
  Relational Operator3 : RelationalOperator  Operator===  OutDataTypeStr=boolean  RndMeth=Nearest
  StreamOut : Outport
  Ctrl : Outport  Port=2
  wires:
  Minus2/1 -> Relational Operator3/2, Relational Operator2/2
  Feature Row Counter/1 -> Relational Operator2/1, Relational Operator3/1, Compare To Zero/1
  Relational Operator2/1 -> Feature Row Counter/1
  Compare To Zero/1 -> Logical Operator/2
  Relational Operator3/1 -> Logical Operator2/1
  Feature_Area/1 -> Minus1/1
  Constant/1 -> Minus1/2
  Logical Operator/1 -> Logical Operator1/1
  Constant1/1 -> Minus2/2
  Feature_Width/1 -> Minus2/1
  Pixel Control Bus Creator/1 -> Ctrl/1
  Delay3/1 -> Feature Area Counter/2, Feature Row Counter/2, Logical Operator5/2, Logical Operator2/2, Logical Operator1/2, Logical Operator3/2, Pixel Control Bus Creator/5
  Stream_In/1 -> Delay35/1
  Logical Operator1/1 -> Pixel Control Bus Creator/1
  Logical Operator2/1 -> Pixel Control Bus Creator/2
  Logical Operator3/1 -> Pixel Control Bus Creator/4
  Logical Operator5/1 -> Pixel Control Bus Creator/3
  Feature Area Counter/1 -> Compare To Zero1/1, Relational Operator1/1
  Minus1/1 -> Relational Operator1/2
  Relational Operator1/1 -> Feature Area Counter/1, Logical Operator3/1
  Compare To Zero1/1 -> Logical Operator/1, Logical Operator5/1
  Delay35/1 -> StreamOut/1
  Stream_Valid/1 -> Delay3/1

== matlab function PE_V2_0/2DCov PEV1.1/MATLAB Function ==
  settings: fimath=fimath('RoundingMethod', 'Floor','OverflowAction', 'Wrap','ProductMode', 'FullPrecision', 'SumMode', 'FullPrecision')
  data: w0 output; dataIn input; w1 output; rst input; write_en input; w2 output; w3 output; w4 output; w5 output; w6 output; w7 output; w8 output
function [w0, w1, w2, w3 , w4, w5, w6, w7, w8] = weight_register(dataIn, rst, write_en)
%#codegen
persistent read_cnt;

% Counter
if(isempty(read_cnt))
   read_cnt = fi(0,1,32,0); 
end

% Max Count = uint32(8)
persistent cntMax;

if(isempty(cntMax))
   cntMax = fi(9 - 1,1,32,0);
end

% weight0
persistent weight0
if(isempty(weight0))
   weight0 = fi(0,1,32,0); 
end

% weight1
persistent weight1
if(isempty(weight1))
   weight1 = fi(0,1,32,0); 
end

% weight2
persistent weight2
if(isempty(weight2))
   weight2 = fi(0,1,32,0); 
end

% weight3
persistent weight3
if(isempty(weight3))
   weight3 = fi(0,1,32,0); 
end

% weight1
persistent weight4
if(isempty(weight4))
   weight4 = fi(0,1,32,0); 
end

% weight5
persistent weight5
if(isempty(weight5))
   weight5 = fi(0,1,32,0); 
end

% weight6
persistent weight6
if(isempty(weight6))
   weight6 = fi(0,1,32,0); 
end

% weight7
persistent weight7
if(isempty(weight7))
   weight7 = fi(0,1,32,0); 
end

% weight8
persistent weight8
if(isempty(weight8))
   weight8 = fi(0,1,32,0); 
end

%%%%%%%%%%%%%%%%%%%%%%%%%%%%%%%%%%%%
% Output Logic
    w0 = weight0;
    w1 = weight1;
    w2 = weight2;
    w3 = weight3;
    w4 = weight4;
    w5 = weight5;
    w6 = weight6;
    w7 = weight7;
    w8 = weight8;
%%%%%%%%%%%%%%%%%%%%%%%%%%%%%%%%%%%%

if (rst == 1)
    % reset the output
    read_cnt = fi(0,1,32,0);
    
    weight0 = fi(0,1,32,0);
    weight1 = fi(0,1,32,0);
    weight2 = fi(0,1,32,0);
    weight3 = fi(0,1,32,0);
    weight4 = fi(0,1,32,0);
    weight5 = fi(0,1,32,0);
    weight6 = fi(0,1,32,0);
    weight7 = fi(0,1,32,0);
    weight8 = fi(0,1,32,0);
elseif (write_en == 1)
    if (read_cnt == cntMax)
        read_cnt = fi(0,1,32,0);
        weight0 = fi(dataIn,1,32,0);
    else
        if (read_cnt == 0)
           weight8 = fi(dataIn,1,32,0);
        elseif (read_cnt == 1)
            weight5 = fi(dataIn,1,32,0);
        elseif (read_cnt == 2)
            weight2 = fi(dataIn,1,32,0);
        elseif (read_cnt == 3)
            weight7 = fi(dataIn,1,32,0);
        elseif (read_cnt == 4)
            weight4 = fi(dataIn,1,32,0);
        elseif (read_cnt == 5)
            weight1 = fi(dataIn,1,32,0);
        elseif (read_cnt == 6)
            weight6 = fi(dataIn,1,32,0);
        elseif (read_cnt == 7)
            weight3 = fi(dataIn,1,32,0);
        end   
        read_cnt = fi(read_cnt+1, 1,32,0);
    end
end
